simulink model "RLcircuit"  (R2018b)
settings: Solver=VariableStepAuto  StartTime=0.0  StopTime=20  RelTol=1e-3
undefined symbols (not defined in the file): E, L, R1, R2
settings Model: Creator=ilab  LastModifiedBy=ilab

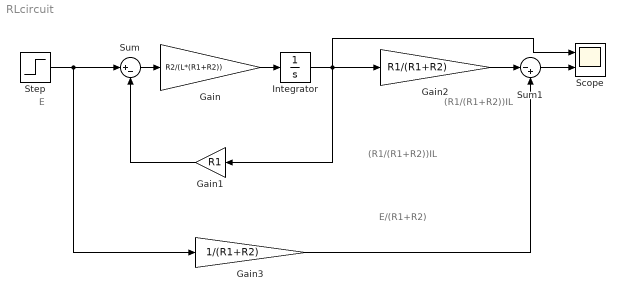
== system RLcircuit ==
  note: (R1/(R1+R2))IL
  note: E
  note: E/(R1+R2)
  note: (R1/(R1+R2))IL
  Gain : Gain  Gain=R2/(L*(R1+R2))
  Gain1 : Gain  Gain=R1
  Gain2 : Gain  Gain=R1/(R1+R2)
  Gain3 : Gain  Gain=1/(R1+R2)
  Integrator : Integrator
  Scope : Scope  NumInputPorts=2
  Step : Step  After=E  SampleTime=0
  Sum : Sum  Inputs=|+-
  Sum1 : Sum  Inputs=|-+
  wires:
  Sum/1 -> Gain/1
  Gain/1 -> Integrator/1
  Step/1 -> Gain3/1, Sum/1
  Gain1/1 -> Sum/2
  Integrator/1 -> Gain2/1, Scope/1, Gain1/1
  Gain2/1 -> Sum1/1
  Sum1/1 -> Scope/2
  Gain3/1 -> Sum1/2
